simulink model "tf_mcp_rotation"  (R2020a)
settings: configuration reference "globalConfig" (kept outside this file)
undefined symbols (not defined in the file): A, B, C, D, magnitude, mcp_nominal_rotation
libraries: simulink_extras x1, cstblocks x1
settings Model: Creator=victo  LastModifiedBy=ToT_IPMS_03
settings ConfigSetRef: SourceName=globalConfig  SourceLocation=Base Workspace

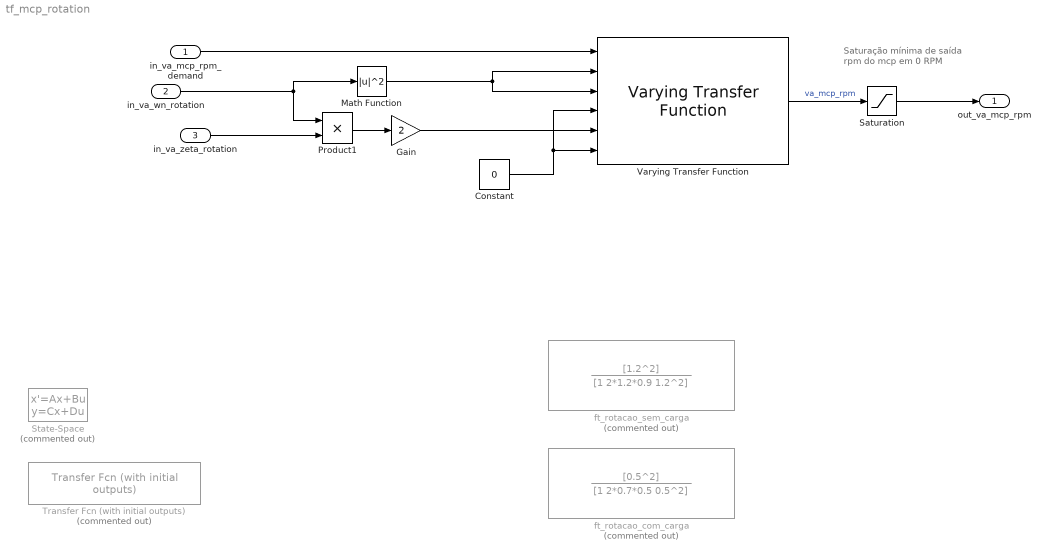
== system tf_mcp_rotation ==
  note: Saturação mínima de saída rpm do mcp em 0 RPM
  in_va_mcp_rpm_demand : Inport  OutMin=[0]  OutMax=[mcp_nominal_rotation]  OutDataTypeStr=uint16  Unit=rpm  PortDimensions=1  SampleTime=0
  in_va_wn_rotation : Inport  Port=2  OutMin=[0.5]  OutMax=[1.2]  OutDataTypeStr=double
  in_va_zeta_rotation : Inport  Port=3  OutMin=[0.7]  OutMax=[0.9]  OutDataTypeStr=double
  Constant : Constant  Value=0
  Gain : Gain  Gain=2
  Math Function : Math  Operator=magnitude^2  SaturateOnIntegerOverflow=on
  Product1 : Product
  Saturation : Saturate  UpperLimit=inf  LowerLimit=0
  State-Space : StateSpace  Commented=on  A=A  B=B  C=C  D=D  InitialCondition=600
  Transfer Fcn (with initial outputs) : simulink_extras/Additional Linear/Transfer Fcn (with initial outputs)  Commented=on  N=[0.0548 0.0518]  D=[1 1.541 0.1773]  Y0=600  U0=600
  Varying Transfer Function : cstblocks/Linear Parameter Varying/Varying Transfer Function  N=2
  ft_rotacao_com_carga : TransferFcn  Commented=on  Numerator=[0.5^2]  Denominator=[1 2*0.7*0.5 0.5^2]
  ft_rotacao_sem_carga : TransferFcn  Commented=on  Numerator=[1.2^2]  Denominator=[1 2*1.2*0.9 1.2^2]
  out_va_mcp_rpm : Outport  OutMin=[0]  OutMax=[2200]
  wires:
  Varying Transfer Function/1 -> Saturation/1  "va_mcp_rpm"
  in_va_mcp_rpm_demand/1 -> Varying Transfer Function/1
  Constant/1 -> Varying Transfer Function/4, Varying Transfer Function/6
  Product1/1 -> Gain/1
  Gain/1 -> Varying Transfer Function/5
  Math Function/1 -> Varying Transfer Function/3, Varying Transfer Function/2
  in_va_zeta_rotation/1 -> Product1/2
  in_va_wn_rotation/1 -> Product1/1, Math Function/1
  Saturation/1 -> out_va_mcp_rpm/1
